simulink model "ppm_psk_shared_v4"  (R2025a)
settings: Solver=VariableStepAuto  StartTime=0.0  StopTime=5e-6  RelTol=1e-3
model workspace (MAT data in the model file):
  Sig = Simulink.Signal
  Sig.Dimensions = -1
  Sig.DimensionsMode = 'auto'
  Sig.Complexity = 'auto'
  Sig.SampleTime = -1
  Sig.SamplingMode = 'auto'
  Sig.DataType = 'auto'
  Var = 0
  fc = 4000000000
  fs = 32000000000
  fsymbol = 500000000
  ppm_spacings2_ps = [-51.8 33.2 115.3 201.3 293.8 377.9 462.9 544.9]
  ppm_spacings_ps = [698 782 869 950 1045 1127 1210 1299]
  up_fs = 1024000000000
libraries: commsink2 x2, simulink_extras x1, dspfdesign x1, commdigbbndpm3 x1, dspsigops x1
settings Model: ParameterArgumentNames=ppm_spacings2_ps,ppm_spacings_ps  Creator=IWMAI  LastModifiedBy=IWMAI

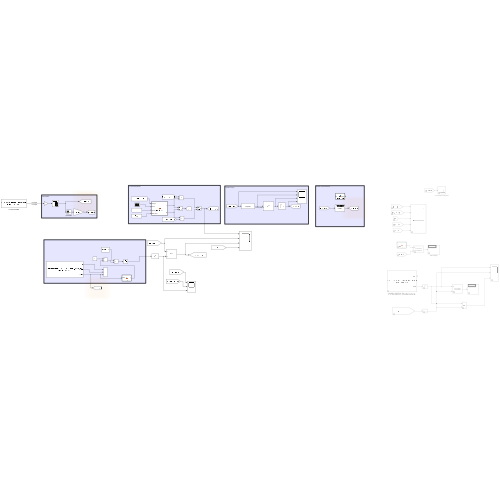
[thumbnail: Simulink's stored preview of the top-level diagram]
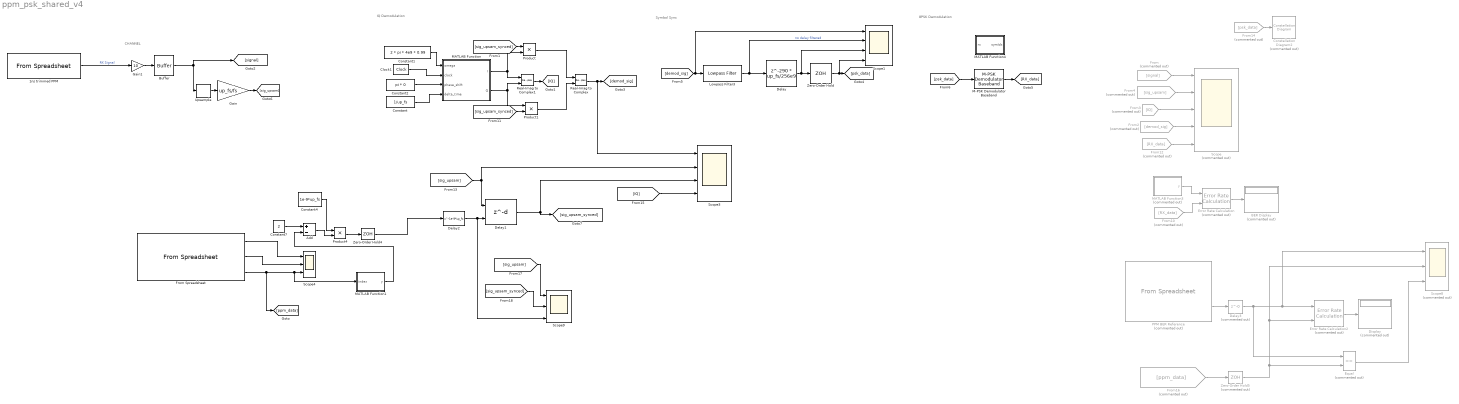
== system ppm_psk_shared_v4 ==
  note: Symbol Sync
  note: IQ Demodulation
  note: 8PSK Demodulation
  note: CHANNEL
  1ns trimmed PPM : FromSpreadsheet  FileName=C:\Users\IWMAI\University of Toronto\Yu Huang - Summer-2025-sharted\Yongkang\v6_250708\csv\phase_noise_ppm32.csv  SheetName=phase_noise_ppm32  SampleTime=1/fs  InterpolationWithinTimeRange=Zero order hold
  Add : Sum  Inputs=+-
  BER Display : Display  Commented=on
  Buffer : Buffer  OutputFrames=off
  Clock1 : simulink_extras/Flip Flops/Clock  period=1/500e6
  Constant : Constant  Value=1/up_fs
  Constant1 : Constant  Value=2 * pi * 4e9 * 0.99
  Constant2 : Constant  Value=pi * 0
  Constant4 : Constant  Value=1e-9*up_fs
  Constant7 : Constant  Value=2
  Constellation Diagram2 : ConstellationDiagram  Commented=on  WindowPosition=[198.000000,182.000000,773.000000,552.000000,]  ScopeFrameLocation=window  SymbolsToDisplaySource=Property  SymbolsToDisplay=2500  ShowLegend=on  MaximizeAxes=on  DefaultConfigurationName=comm.scopes.ConstellationDiagramBlockCfg
  Delay : Delay  DelayLength=290 * up_fs/256e9  DelayLengthUpperLimit=512  InputProcessing=Columns as channels (frame based)
  Delay1 : Delay  DelayLengthSource=Input port  DelayLength=1  DelayLengthUpperLimit=2*up_fs/1e9  InputProcessing=Columns as channels (frame based)
      settings: InputPortMap=u0,p1
  Delay2 : Delay  DelayLength=1e-9*up_fs
  Delay3 : Delay  Commented=on  DelayLength=0
  Display : Display  Commented=on
  Equal : RelationalOperator  Commented=on  Operator===  OutDataTypeStr=boolean  RndMeth=Simplest  InputSameDT=off
  Error Rate Calculation : commsink2/Error Rate Calculation  Commented=on  N=0  st_delay=0  cp_mode=Entire frame  subframe=[]  PMode=Port  WsName=ErrorVec  RsMode2=off  stop=off  numErr=100  maxBits=1e6
      settings: LibrarySourceBlock=|
      | commhdlsink/Error Rate
      | Calculation
  Error Rate Calculation2 : commsink2/Error Rate Calculation  Commented=on  N=0  st_delay=0  cp_mode=Entire frame  subframe=[]  PMode=Port  WsName=ErrorVec  RsMode2=off  stop=off  numErr=100  maxBits=1e6
      settings: LibrarySourceBlock=|
      | commhdlsink/Error Rate
      | Calculation
  From : From  Commented=on  GotoTag=signal
  From Spreadsheet : FromSpreadsheet  FileName=C:\Users\IWMAI\University of Toronto\Yu Huang - Summer-2025-sharted\Yongkang\v6_250708\csv\ppm_decode_1024.csv  SheetName=ppm_decode_1024  TreatFirstColumnAs=Data  SampleTime=1/fsymbol
  From10 : From  Commented=on  GotoTag=RX_data
  From12 : From  Commented=on  GotoTag=RX_data
  From14 : From  Commented=on  GotoTag=psk_data
  From16 : From  Commented=on  GotoTag=ppm_data
  From2 : From  Commented=on  GotoTag=demod_sig
  From3 : From  Commented=on  GotoTag=IQ
  From4 : From  Commented=on  GotoTag=sig_upsam
  Gain : Gain  Gain=up_fs/fs
  Gain1 : Gain  Gain=10
  Lowpass Filter3 : dspfdesign/Lowpass Filter  FilterType=FIR  DesignForMinimumOrder=on  FilterOrder=50  PassbandFrequency=0.05*fc  StopbandFrequency=0.6*fc  PassbandRipple=0.1  StopbandAttenuation=80  SampleRate=fs  SimulateUsing=Interpreted execution  roundingMode=Floor  coeffsDataTypeStr=fixdt(1,16)
  M-PSK Demodulator Baseband : commdigbbndpm3/M-PSK Demodulator Baseband  M=8  OutType=Integer  DecType=Hard decision  VarSource=Dialog  Variance=1  Dec=Gray  Mapping=[0:7]  Ph=pi/8  outDtype1=Inherit via internal rule  outDtype2=Inherit via internal rule  derotateFactorWordLen=16  derotateFactorDataTypeStr=Inherit: Same word length as input  derotateFactorLastDataTypeStr=Inherit: Same word length as input
      settings: LibrarySourceBlock=|
      | commhdldigbbndpm/M-PSK
      | Demodulator
      | Baseband
  MATLAB Function : MATLAB Function  TreatAsAtomicUnit=on  SystemSampleTime=1/up_fs
  MATLAB Function1 : MATLAB Function  TreatAsAtomicUnit=on
  MATLAB Function3 : MATLAB Function  Commented=on  TreatAsAtomicUnit=on  SystemSampleTime=1/500e6
  MATLAB Function4 : MATLAB Function  TreatAsAtomicUnit=on
  PPM BER Reference : FromSpreadsheet  Commented=on  FileName=C:\Users\IWMAI\University of Toronto\Yu Huang - Summer-2025-sharted\Yongkang\v5_250626\csv\ground_truth_ppm.csv  SheetName=ground_truth_ppm  TreatFirstColumnAs=Data  SampleTime=1/fsymbol
  Product : Product
  Product1 : Product
  Product4 : Product
  Real-Imag to Complex : RealImagToComplex
  Real-Imag to Complex1 : RealImagToComplex
  Scope : Scope  Commented=on  NumInputPorts=5
      settings: ActiveDisplayYMinimum=-3.2971710288295304  ActiveDisplayYMaximum=3.6439303524490732
  Scope1 : Scope  NumInputPorts=4
      settings: ActiveDisplayYMinimum=-217.12328360095091  ActiveDisplayYMaximum=190.25679951109339  DataLoggingVariableName=ScopeData3
  Scope3 : Scope  NumInputPorts=4
      settings: ActiveDisplayYMinimum=-121.24929806481079  ActiveDisplayYMaximum=113.85916593857471  DataLoggingVariableName=ScopeData11
  Scope4 : Scope  NumInputPorts=3
      settings: ActiveDisplayYMinimum=-62.374999999999986  ActiveDisplayYMaximum=561.375  DataLoggingVariableName=ScopeData13
  Scope8 : Scope  Commented=on  NumInputPorts=3
      settings: ActiveDisplayYMinimum=-0.87499999999999978  ActiveDisplayYMaximum=7.875  DataLoggingVariableName=ScopeData17
  Scope9 : Scope  NumInputPorts=3
      settings: ActiveDisplayYMinimum=-2041.2616026203843  ActiveDisplayYMaximum=448.10816733090951  DataLoggingVariableName=ScopeData18
  Upsample : dspsigops/Upsample  FactorSource=Dialog parameter  N=up_fs/fs  Nmax=16  phase=0  RateOptions=Allow multirate processing  ic=0  mode=Unused parameter value
      settings: LibrarySourceBlock=dsphdlsupportsigops/Upsample
  Zero-Order Hold : ZeroOrderHold  SampleTime=1/fsymbol
  Zero-Order Hold4 : ZeroOrderHold  SampleTime=1/up_fs
  Zero-Order Hold5 : ZeroOrderHold  Commented=on  SampleTime=1/fsymbol
  wires:
  MATLAB Function3/1(y) -> Error Rate Calculation/1
  Error Rate Calculation/1 -> BER Display/1
  From/1 -> Scope/1
  From3/1 -> Scope/3
  [demod_sig] -> Scope1/1, Lowpass Filter3/1
  Zero-Order Hold/1 -> Scope1/4, [psk_data]
  [psk_data] -> M-PSK Demodulator Baseband/1
  M-PSK Demodulator Baseband/1 -> [RX_data]
  From10/1 -> Error Rate Calculation/2
  Real-Imag to Complex1/1 -> [IQ]
  Constant1/1 -> MATLAB Function/1(omega)
  Clock1/1 -> MATLAB Function/2(clock)
  Constant2/1 -> MATLAB Function/3(phase_shift)
  MATLAB Function/1(I) -> Real-Imag to Complex1/1, Product/2
  MATLAB Function/2(Q) -> Product1/1, Real-Imag to Complex1/2
  [sig_upsam_synced] -> Product/1
  [sig_upsam_synced] -> Product1/2
  Product/1 -> Real-Imag to Complex/1
  Product1/1 -> Real-Imag to Complex/2
  Real-Imag to Complex/1 -> Scope3/1, [demod_sig]
  From2/1 -> Scope/4
  From12/1 -> Scope/5
  1ns trimmed PPM/1 -> Gain1/1  "RX Signal"
  Gain1/1 -> Buffer/1
  Constant/1 -> MATLAB Function/4(delta_time)
  Lowpass Filter3/1 -> Scope1/2, Delay/1  "no delay filtered"
  Upsample/1 -> Gain/1
  From4/1 -> Scope/2
  From Spreadsheet/1 -> Scope4/1
  From Spreadsheet/2 -> Scope4/2
  From Spreadsheet/3 -> [ppm_data], MATLAB Function1/1(index), Scope4/3
  Constant4/1 -> Product4/1
  Constant7/1 -> Add/1
  Add/1 -> Product4/2
  Delay/1 -> Scope1/3, Zero-Order Hold/1
  Product4/1 -> Zero-Order Hold4/1
  [sig_upsam] -> Delay1/1, Scope3/2
  Delay1/1 -> [sig_upsam_synced], Scope3/3
  Zero-Order Hold4/1 -> Delay2/1
  Delay2/1 -> Scope9/3, Delay1/2
  From14/1 -> Constellation Diagram2/1
  Gain/1 -> [sig_upsam]
  [IQ] -> Scope3/4
  PPM BER Reference/2 -> Delay3/1
  Equal/1 -> Scope8/3
  Error Rate Calculation2/1 -> Display/1
  Zero-Order Hold5/1 -> Scope8/2, Error Rate Calculation2/2, Equal/2
  Delay3/1 -> Scope8/1, Error Rate Calculation2/1, Equal/1
  From16/1 -> Zero-Order Hold5/1
  [sig_upsam] -> Scope9/1
  [sig_upsam_synced] -> Scope9/2
  MATLAB Function1/1(y) -> Add/2
  Buffer/1 -> [signal], Upsample/1

== matlab function ppm_psk_shared_v4/MATLAB Function1 ==
  data: index input; y output
function y = mapp(index)

map = [0.6943 0.7793 0.8663 0.9512 1.0423 1.1270 1.2079 1.2933];
map2 = [0.6922 0.7774 0.8653 0.9521 1.0420 1.1250 1.2061 1.2891];
map3 = [0.6758 0.7578 0.8474 0.9297 1.0129 1.1010 1.1836 1.2695];
map4 = [0.6769 0.7575 0.8466 0.9310 1.0135 1.1012 1.1848 1.2694];
map5 = [0.67187500 0.75683594 0.84277344 0.92773438 1.01269531 1.09808077 1.18359375 1.26793381];
map6 = [0.67187500 0.75683594 0.84277344 0.92773438 1.01269531 1.09850530 1.18359375 1.26828013];

y = map6(index + 1);

== matlab function ppm_psk_shared_v4/MATLAB Function ==
  data: omega input; clock input; I output; phase_shift input; Q output; delta_time input
function [I, Q]= custom_sine(omega, clock, phase_shift, delta_time)

% around 4GHz sine wave, restart 1/500e6 sec
% currently assume the sample rate is 16S/s

persistent count;
persistent last_clock; % for detecting the falling edge, because we want to reset the wave on the falling edge

if isempty(count)
    count = 0;
    last_clock = 1;
end

if clock == 0 && last_clock == 1 % means we are on a falling edge
    count = 0;
end

phase = count * omega * delta_time + phase_shift;

I = cos(phase);
Q = -sin(phase);

count = count + 1;
last_clock = clock;

== matlab function ppm_psk_shared_v4/MATLAB Function3 ==
  data: y output
function y = TX_data

persistent index;
persistent ans_buffer;

buffer_len = 127;

if isempty(index)
    index = 1;
    ans_buffer = [7 4 2 2 2 2 2 6 5 3 3 3 3 7 2 7 5 5 5 1 0 2 1 7 7 3 6 7 0 5 3 7 6 4 4 0 7 1 4 1 7 3 6 7 4 6 5 7 6 4 0 3 4 5 6 3 5 4 2 2 2 6 1 2 7 5 5 1 0 6 2 1 7 3 6 3 5 0 5 7 6 0 3 0 2 5 6 7 4 6 1 6 4 4 0 3 0 2 1 7 3 2 4 7 0 5 7 2 3 0 6 2 5 2 0 4 3 5 4 6 5 7 2 3 4 5 6];
end

y = ans_buffer(mod(index, buffer_len) + 1);
index = index + 1;

== matlab function ppm_psk_shared_v4/MATLAB Function4 ==
  data: rx input; symIdx output
function symIdx = my_8psk_decoder(rx)
% rx: complex input symbol
% symIdx: integer index [0~7]

% 固定参考点（从 Python 得到）
persistent centers
if isempty(centers)
    centers = [
-0.794546 + -0.298444i;
-0.425530 + -0.703649i;
0.731182 + -0.125290i;
0.232761 + -0.730665i;
-0.220880 + 0.731179i;
-0.772253 + 0.362395i;
0.270349 + 0.746917i;
0.682762 + 0.402678i;
    ]; % 改成你实际的
end

% 最小距离判决
dist = abs(rx - centers);
[~, symIdx] = min(dist);

symIdx = symIdx - 1; % MATLAB index从1开始，转成0~7
